simulink model "lista1_11"  (R2020a)
settings: Solver=FixedStepAuto  StartTime=0.0  StopTime=50  FixedStep=0.001  RelTol=1e-3
settings Model: Creator=bruno  LastModifiedBy=bruno

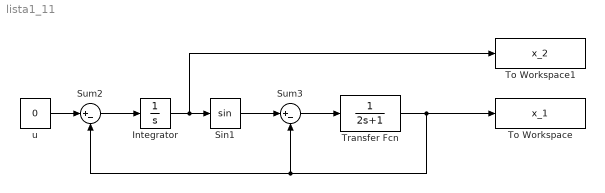
== system lista1_11 ==
  Integrator : Integrator  InitialCondition=pi - pi/2
  Sin1 : Trigonometry
  Sum2 : Sum  Inputs=|+-
  Sum3 : Sum  Inputs=|+-
  To Workspace : ToWorkspace  VariableName=x_1  SaveFormat=Timeseries  SampleTime=-1
  To Workspace1 : ToWorkspace  VariableName=x_2  SaveFormat=Timeseries  SampleTime=-1
  Transfer Fcn : TransferFcn  Denominator=[2 1]
  u : Constant  Value=0
  wires:
  u/1 -> Sum2/1
  Sum2/1 -> Integrator/1
  Integrator/1 -> To Workspace1/1, Sin1/1
  Sin1/1 -> Sum3/1
  Sum3/1 -> Transfer Fcn/1
  Transfer Fcn/1 -> Sum2/2, Sum3/2, To Workspace/1
